simulink model "BPSK_mod"  (R2023b)
settings: Solver=VariableStepAuto  StartTime=0.0  StopTime=10.0  RelTol=1e-3
settings Model: Creator=adiicmp_  LastModifiedBy=adiicmp_

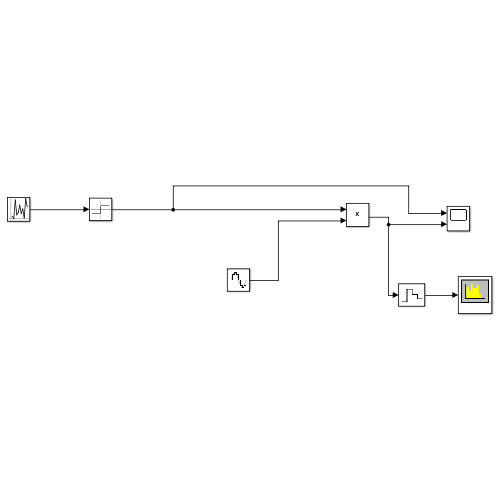
[thumbnail: Simulink's stored preview of the top-level diagram]
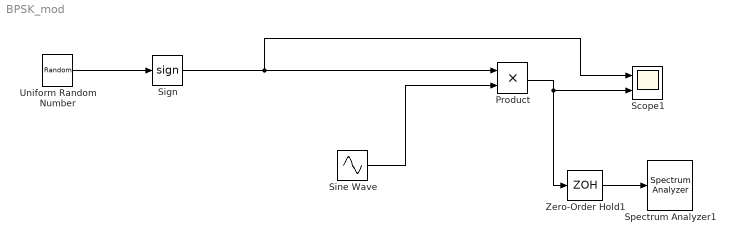
== system BPSK_mod ==
  Product : Product
  Scope1 : Scope  NumInputPorts=2
  Sign : Signum
  Sine Wave : Sin  SampleTime=0.01
  Spectrum Analyzer1 : SpectrumAnalyzer  WindowPosition=[440.000000,275.000000,800.000000,500.000000,]  ScopeFrameLocation=window
  Uniform Random Number : UniformRandomNumber  SampleTime=0.01
  Zero-Order Hold1 : ZeroOrderHold  SampleTime=-1
  wires:
  Uniform Random Number/1 -> Sign/1
  Product/1 -> Zero-Order Hold1/1, Scope1/2
  Zero-Order Hold1/1 -> Spectrum Analyzer1/1
  Sine Wave/1 -> Product/2
  Sign/1 -> Scope1/1, Product/1
